simulink model "nomoto_1st"  (R2016a)
settings: Solver=VariableStepAuto  StartTime=0.0  StopTime=30  MaxStep=1e-2  RelTol=1e-3
values from neighbouring files (symbols this model uses):
  K = linspace(-5,5,N)    [drone_folowing_A.m]    (also in nomoto_1st_Kp_init.m = -0.2; nomoto_1st_init.m = -0.2; nomoto_1st_stability.m = -0.2)
  T = 16.4    [nomoto_1st_Kp_init.m]    (also in nomoto_1st_init.m; nomoto_1st_stability.m)
undefined symbols (not defined in the file or in its folder): step
settings Model: Creator=alexalcocer  LastModifiedBy=alepen

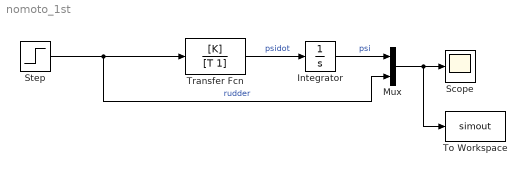
== system nomoto_1st ==
  Integrator : Integrator
  Mux : Mux  Inputs=2
  Scope : Scope
  Step : Step  Time=step.time  After=step.value  SampleTime=0
  To Workspace : ToWorkspace  VariableName=simout  SaveFormat=Timeseries  SampleTime=-1
  Transfer Fcn : TransferFcn  Numerator=[K]  Denominator=[T 1]
  wires:
  Mux/1 -> To Workspace/1, Scope/1
  Step/1 -> Transfer Fcn/1, Mux/2  "rudder"
  Transfer Fcn/1 -> Integrator/1  "psidot"
  Integrator/1 -> Mux/1  "psi"
